simulink model "Verifica_EIG"  (R2025b)
settings: Solver=VariableStepAuto  StartTime=0.0  StopTime=10.0  RelTol=1e-3
values from neighbouring files (symbols this model uses):
  A = double(subs(A_sym, x, x_star))    [SvolgimentoEsame_11032026.m]
  B = double(subs(B_sym, x, x_star))    [SvolgimentoEsame_11032026.m]
  C = eye(4)    [SvolgimentoEsame_11032026.m]
  N = -inv(C_N * (A_cl \ B))    [SvolgimentoEsame_11032026.m]
undefined symbols (not defined in the file or in its folder): C_eig, D_eig, K_EIG, q0, q_ref
settings Model: Creator=salvo  LastModifiedBy=salvo

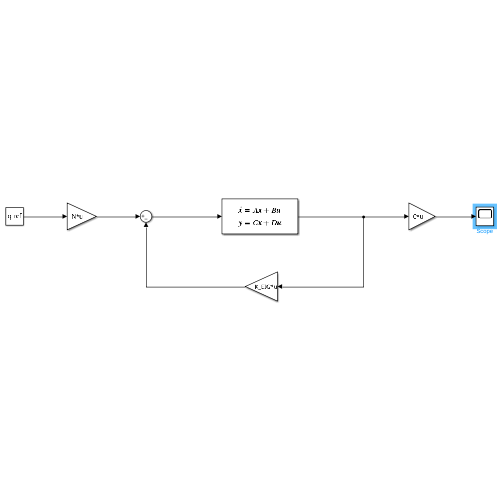
[thumbnail: Simulink's stored preview of the top-level diagram]
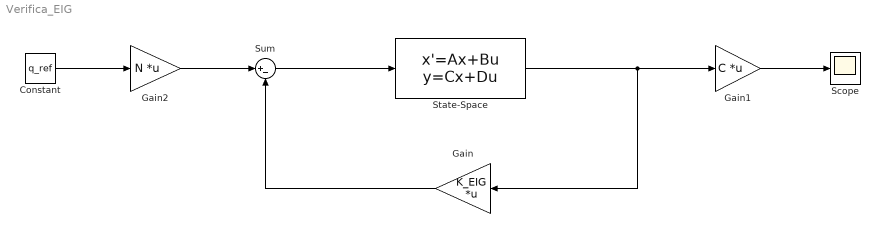
== system Verifica_EIG ==
  Constant : Constant  Value=q_ref
  Gain : Gain  Gain=K_EIG  Multiplication=Matrix(K*u)
  Gain1 : Gain  Gain=C  Multiplication=Matrix(K*u)
  Gain2 : Gain  Gain=N  Multiplication=Matrix(K*u)
  Scope : Scope
      settings: ActiveDisplayYMinimum=-0.4264046857096363  ActiveDisplayYMaximum=1.4816872815242714
  State-Space : StateSpace  A=A  B=B  C=C_eig  D=D_eig  InitialCondition=q0
  Sum : Sum  Inputs=|+-
  wires:
  Sum/1 -> State-Space/1
  Gain/1 -> Sum/2
  State-Space/1 -> Gain1/1, Gain/1
  Gain1/1 -> Scope/1
  Constant/1 -> Gain2/1
  Gain2/1 -> Sum/1
